simulink library "sm_wheel_loader_lib"  (R2026a)
settings: Solver=VariableStepAuto
undefined symbols (not defined in the file): AToTOrificeVector, BiPOrificeVector, boomHEArea, boomREArea, BToTOrificeVector, fluids, GRake, GToothL, GToothR, HMPST, HydFcnParams, logLoad, Position, PToAOrificeVector, PToBOrificeVector, RakeL, RakeR, testInput, Wheel_Loader, X, Y, Z
libraries: sm_lib x694, fl_lib x183, nesl_utility x74, SimscapeFluids_lib x62, sdl_lib x25, cvt_components_lib x25, simulink_extras x5, $bdroot x4, wheel_loader_contact_lib x4, ee_lib x2, SignalEditorBlockLib x1, batteryecm_lib x1
(part 3 of 25)

== system sm_wheel_loader_lib/CVT Power Split Hydromechanical/Hydrostatic ==
  Ctrl : Inport
  CV Charge Pump : fl_lib/Isothermal Liquid/Elements/Constant Volume Chamber (IL)  volume=1e-4 m^3  p_I_specify=off  p_I_priority=High  p_I=0.101325 MPa  p_I_nominal_specify=off  p_I_nominal_value=1  p_I_nominal_unit=MPa
  CV Motor A : fl_lib/Isothermal Liquid/Elements/Constant Volume Chamber (IL)  volume=1e-4 m^3  p_I_specify=off  p_I_priority=High  p_I=0.101325 MPa  p_I_nominal_specify=off  p_I_nominal_value=1  p_I_nominal_unit=MPa
  CV Motor B : fl_lib/Isothermal Liquid/Elements/Constant Volume Chamber (IL)  volume=1e-4 m^3  p_I_specify=off  p_I_priority=High  p_I=0.101325 MPa  p_I_nominal_specify=off  p_I_nominal_value=1  p_I_nominal_unit=MPa
  CV Pump A : fl_lib/Isothermal Liquid/Elements/Constant Volume Chamber (IL)  volume=1e-4 m^3  p_I_specify=off  p_I_priority=High  p_I=0.101325 MPa  p_I_nominal_specify=off  p_I_nominal_value=1  p_I_nominal_unit=MPa
  CV Pump B : fl_lib/Isothermal Liquid/Elements/Constant Volume Chamber (IL)  volume=1e-4 m^3  p_I_specify=off  p_I_priority=High  p_I=0.101325 MPa  p_I_nominal_specify=off  p_I_nominal_value=1  p_I_nominal_unit=MPa
  Charge Pump : Subsystem  Tag=PublishSubsystem  mask{chgPumpNomDisp=chgPumpNomDisp, chgPumpNomSpd=chgPumpNomSpd, chgPumpNomPressGain=chgPumpNomPressGain, chgPumpNomVolEff=chgPumpNomVolEff, chgPumpNomMechEff=chgPumpNomMechEff, chgPumpChkvPdiff=chgPumpChkvPdiff, chgPumpChkvPrange=chgPumpChkvPrange, chgPumpChkvAmax=chgPumpChkvAmax, chgPumpChkvAleak=chgPumpChkvAleak}
      mask prompts: chgPumpNomDisp "Displacement (cm^3/rev)"; chgPumpNomSpd "Nominal Angular Velocity (rpm)"; chgPumpNomPressGain "Nominal pressure gain (MPa)"; chgPumpNomVolEff "Nominal Volumetric Efficiency (0-1)"; chgPumpNomMechEff "Nominal Mechanical Efficiency (0-1)"; chgPumpChkvPdiff "Set pressure differential (MPa)"; chgPumpChkvPrange "Pressure regulation range (MPa)"; chgPumpChkvAmax "Maximum opening area (m^2)"; chgPumpChkvAleak "Leakage area (m^2)"
      mask TypeOptions chgPumpNomDisp: Pump/displacement
      mask TypeOptions chgPumpNomSpd: Pump/omega_nominal
      mask TypeOptions chgPumpNomPressGain: Pump/p_nominal
      mask TypeOptions chgPumpNomVolEff: Pump/vol_eff_nominal
      mask TypeOptions chgPumpNomMechEff: Pump/mech_eff_nominal
      mask TypeOptions chgPumpChkvPdiff:
      | Pressure
      | Relief
      | Valve/p_set_differential
      mask TypeOptions chgPumpChkvPrange:
      | Pressure
      | Relief
      | Valve/p_range
      mask TypeOptions chgPumpChkvAmax:
      | Pressure
      | Relief
      | Valve/area_max
      mask TypeOptions chgPumpChkvAleak:
      | Pressure
      | Relief
      | Valve/area_leak
      mask DialogControl grp_chg_pump Prompt: Pump
      mask DialogControl grp_chg_pump_prv Prompt: Pressure Relief Valve
      mask Display:
      | % Circle
      | color('green')
      | plot(2*cos(linspace(0, 2*pi, 100)), 2*sin(linspace(0, 2*pi, 100)))
      | % Triangle
      | patch([1 0.4 0.4]*2, [0,-0.4,0.4]*2,[45 48 173]/255)
      | % Boundary
      | color('white')
      | plot(-2, -2)
      | plot(2, 2)
  Check Valve A : SimscapeFluids_lib/Isothermal Liquid/Valves & Orifices/Directional Control Valves/Check Valve (IL)  opening_spec=2*(fluids.isothermal_liquid.valves_orifices.enum.PressureOpeningSpec.Linear)-1  pressure_control_spec=fluids.isothermal_liquid.valves_orifices.enum.pressure_control_spec.dp  p_crack_differential=p_crack_differential MPa  p_crack_gauge=0.1 MPa  press_max_differential=press_max_differential MPa  press_max_gauge=0.2 MPa  area_max=chkv_area_max m^2  area_leak=chkv_area_leak m^2  p_diff_TLU=[0.01 : 0.01 : 0.1] MPa  valve_area_TLU=[1e-10, 1e-05, 2e-05, 3e-05, 4e-05, 5e-05, 6e-05, 7.5e-05, 8.5e-05, .0001] m^2  vol_flow_TLU=[.000358, .045, .11, .191, .284, .39, .505, .63, .764, .905] .* 1e-3 m^3/s  area=inf m^2  Cd=0.64  Re_c=150  smoothing_factor=0.01  pressure_recovery=simscape.enum.onoff.off  opening_dynamics=simscape.enum.onoff.off  tau=0.1 s
  Check Valve B : SimscapeFluids_lib/Isothermal Liquid/Valves & Orifices/Directional Control Valves/Check Valve (IL)  opening_spec=2*(fluids.isothermal_liquid.valves_orifices.enum.PressureOpeningSpec.Linear)-1  pressure_control_spec=fluids.isothermal_liquid.valves_orifices.enum.pressure_control_spec.dp  p_crack_differential=p_crack_differential MPa  p_crack_gauge=0.1 MPa  press_max_differential=press_max_differential MPa  press_max_gauge=0.2 MPa  area_max=chkv_area_max m^2  area_leak=chkv_area_leak m^2  p_diff_TLU=[0.01 : 0.01 : 0.1] MPa  valve_area_TLU=[1e-10, 1e-05, 2e-05, 3e-05, 4e-05, 5e-05, 6e-05, 7.5e-05, 8.5e-05, .0001] m^2  vol_flow_TLU=[.000358, .045, .11, .191, .284, .39, .505, .63, .764, .905] .* 1e-3 m^3/s  area=inf m^2  Cd=0.64  Re_c=150  smoothing_factor=0.01  pressure_recovery=simscape.enum.onoff.off  opening_dynamics=simscape.enum.onoff.off  tau=0.1 s
  Gain1 : Gain  Gain=pumpNomDisp
  Gain2 : Gain  Gain=-1
  Mechanical Rotational Reference : fl_lib/Mechanical/Rotational Elements/Mechanical Rotational Reference
  Mechanical Rotational Reference1 : fl_lib/Mechanical/Rotational Elements/Mechanical Rotational Reference
  Motor : SimscapeFluids_lib/Isothermal Liquid/Pumps & Motors/Fixed-Displacement Motor (IL)  leakage_friction_spec=fluids.isothermal_liquid.pumps_motors.enum.MotorLossSpec.Analytical  displacement=motorNomDisp cm^3/rev  omega_nominal=motorNomSpd rpm  p_nominal=motorNomPressDrop MPa  vol_eff_nominal=motorNomVolEff  mech_eff_nominal=motorNomMechEff  no_load_torque=0 N*m  p_diff_eff_TLU=[.1, 1, 2] MPa  omega_eff_TLU=[25, 50, 100, 200, 300, 400] rad/s  vol_eff_TLU=[.816, .908, .954, .977, .981, .984; .325, .663, .831, .916, .925, .946; .137, .568, .78, .892, .893, .91]  mech_eff_TLU=[.996, .996, .996, .996, .996, .996; .988, .989, .989, .989, .989, .99; .981, .981, .982, .982, .983, .984]  p_diff_loss_TLU=[.1, 1, 2] MPa  omega_loss_TLU=[25, 50, 100, 200, 300, 400] rad/s  vol_loss_TLU=[.023, .023, .023, .023, .0285, .032; .0844, .0842, .0845, .084, .1125, .108; .1079, .108, .11, .108, .1605, .18] * 1e-3 m^3/s  mech_loss_TLU=[.002, .002, .002, .002, .002, .002; .0607, .0556, .0556, .0556, .0556, .0505; .1937, .1937, .1833, .1833, .1729, .1626] N*m  q_shaft_TLU=[.125, .25, .5, 1, 1.5, 2] * 1e-3 m^3/s  p_diff_shaft_TLU=[.1, 1, 2] MPa  torque_shaft_TLU=[.47, 4.72, 9.35; .47, 4.7, 9.36; .47, 4.7, 9.4; .47, 4.7, 9.41; .47, 4.7, 9.46; .47, 4.68, 9.5] N*m  omega_shaft_TLU=[205, 80, 35; 455, 330, 285; 955, 831, 780; 1950, 1830, 1780; 2940, 2775, 2680; 3940, 3780, 3640] rpm  vol_eff_min=1e-3  vol_eff_max=1  mech_eff_min=1e-3  mech_eff_max=1  pressure_threshold=1e-3 MPa  omega_threshold=10 rad/s  supplied_range_check=simscape.enum.assert.action.none  motor_mode_check=simscape.enum.assert.action.none  pressure_check=simscape.enum.assert.action.none  p_min_valid=0.101325 MPa
  Motor Leakage : Subsystem  Tag=PublishSubsystem
  "Pipe A " : fl_lib/Isothermal Liquid/Elements/Pipe (IL)  length=pipeLen m  area=pipeAreaGeo m^2  Dh=pipeAreaHydr m  length_add=4 m  roughness=15e-6 m  Re_lam=2000  Re_tur=4000  shape_factor=64  dynamic_compressibility=simscape.enum.onoff.on  inertia=simscape.enum.onoff.off  p0=0.101325 MPa  mdot0=0 kg/s
  Pipe B : fl_lib/Isothermal Liquid/Elements/Pipe (IL)  length=pipeLen m  area=pipeAreaGeo m^2  Dh=pipeAreaHydr m  length_add=4 m  roughness=15e-6 m  Re_lam=2000  Re_tur=4000  shape_factor=64  dynamic_compressibility=simscape.enum.onoff.on  inertia=simscape.enum.onoff.off  p0=0.101325 MPa  mdot0=0 kg/s
  Pressure Relief Valve A : SimscapeFluids_lib/Isothermal Liquid/Valves & Orifices/Pressure Control Valves/Pressure Relief Valve (IL)  set_pressure_spec=foundation.enum.constant_controlled.constant  opening_spec=fluids.isothermal_liquid.valves_orifices.enum.opening_spec.linear  pressure_spec=fluids.isothermal_liquid.valves_orifices.enum.pressure_control_spec.dp  p_set_gauge=0.1 MPa  p_set_differential=p_set_differential MPa  p_range=p_range MPa  area_max=prv_area_max m^2  area_leak=prv_area_leak m^2  p_diff_TLU=[0.2 : 0.2 : 1.2] MPa  p_gauge_TLU=[0.2 : 0.2 : 1.2] MPa  valve_area_TLU=[1e-10, 2e-06, 4e-06, 6e-06, 8e-06, 1e-05] m^2  vol_flow_TLU=[1e-09, 3.6e-05, 8.9e-05, .00015, .00023, .00031] m^3/s  area=inf m^2  Cd=0.64  Re_c=150  smoothing_factor=0.01  pressure_recovery=simscape.enum.onoff.off  opening_dynamics=simscape.enum.onoff.off  tau=0.1 s
  Pressure Relief Valve B : SimscapeFluids_lib/Isothermal Liquid/Valves & Orifices/Pressure Control Valves/Pressure Relief Valve (IL)  set_pressure_spec=foundation.enum.constant_controlled.constant  opening_spec=fluids.isothermal_liquid.valves_orifices.enum.opening_spec.linear  pressure_spec=fluids.isothermal_liquid.valves_orifices.enum.pressure_control_spec.dp  p_set_gauge=0.1 MPa  p_set_differential=p_set_differential MPa  p_range=p_range MPa  area_max=prv_area_max m^2  area_leak=prv_area_leak m^2  p_diff_TLU=[0.2 : 0.2 : 1.2] MPa  p_gauge_TLU=[0.2 : 0.2 : 1.2] MPa  valve_area_TLU=[1e-10, 2e-06, 4e-06, 6e-06, 8e-06, 1e-05] m^2  vol_flow_TLU=[1e-09, 3.6e-05, 8.9e-05, .00015, .00023, .00031] m^3/s  area=inf m^2  Cd=0.64  Re_c=150  smoothing_factor=0.01  pressure_recovery=simscape.enum.onoff.off  opening_dynamics=simscape.enum.onoff.off  tau=0.1 s
  Pump : SimscapeFluids_lib/Isothermal Liquid/Pumps & Motors/Variable-Displacement Pump (IL)  leakage_friction_spec=fluids.isothermal_liquid.pumps_motors.enum.pump_motor_loss_spec.analytical  displacement_nominal=pumpNomDisp cm^3/rev  omega_nominal=pumpNomSpd rpm  p_nominal=pumpNomPressGain MPa  vol_eff_nominal=pumpNomVolEff  mech_eff_nominal=pumpNomMechEff  no_load_torque=0 N*m  p_diff_eff_TLU=[.1, 1, 2] MPa  omega_eff_TLU=[25, 50, 100, 200, 300, 400] rad/s  displacement_eff_TLU=[-30, -19, 19, 30] cm^3/rev  vol_eff_TLU=repmat([.816, .908, .954, .977, .981, .984; .325, .663, .831, .916, .925, .946; .137, .568, .78, .892, .893, .91], 1, 1, 4)  mech_eff_TLU=repmat([.996, .996, .996, .996, .996, .996; .988, .989, .989, .989, .989, .99; .981, .981, .982, .982, .983, .984], 1, 1, 4)  p_diff_loss_TLU=[.1, 1, 2] MPa  omega_loss_TLU=[25, 50, 100, 200, 300, 400] rad/s  displacement_loss_TLU=[-30, -19, 19, 30] cm^3/rev  vol_loss_TLU=repmat([.023, .023, .023, .023, .0285, .032; .0844, .0842, .0845, .084, .1125, .108; .1079, .108, .11, .108, .1605, .18] * 1e-3, 1, 1, 4) m^3/s  mech_loss_TLU=repmat([.002, .002, .002, .002, .002, .002; .0607, .0556, .0556, .0556, .0556, .0505; .1937, .1937, .1833, .1833, .1729, .1626], 1, 1, 4) N*m  vol_eff_min=1e-3  vol_eff_max=1  mech_eff_min=1e-3  mech_eff_max=1  pressure_threshold=1e-3 MPa  omega_threshold=10 rad/s  displacement_threshold=0.1 cm^3/rev  supplied_range_check=simscape.enum.assert.action.none  pump_mode_check=simscape.enum.assert.action.none  pressure_check=simscape.enum.assert.action.none  p_min_valid=0.101325 MPa
  Pump Leakage : Subsystem  Tag=PublishSubsystem
  Simulink-PS Converter1 : nesl_utility/Simulink-PS Converter  PhysicalDomain=network_engine_domain  SubClassName=ps_input  LeftPortType=input  RightPortType=output  PseudoPeriodic=off  Frequencies=[]  NoiseDistribution=none  NoiseParameters=[]  Unit=cm^3/rev  AffineConversion=off  FilteringAndDerivatives=provide  SimscapeFilterOrder=1  InputFilterTimeConstant=0.001  UdotUserProvided=0
  Transmission Fluid Properties : fl_lib/Isothermal Liquid/Utilities/Isothermal Liquid Properties (IL)  rho_L_atm=850 kg/m^3  bulk_modulus_model=foundation.enum.bulk_modulus_model.const  beta_gain=6  beta_L_atm=1.4 GPa  nu_atm=18.8 cSt  p_atm=0.101325 MPa  p_min=0.1 Pa  properties_range_check=simscape.enum.assert.action.error  air_fraction=0.005  polytropic_index=1.0  rho_g_atm=1.225 kg/m^3  air_dissolution_model=simscape.enum.onoff.off  p_crit=3 MPa
  In : PMIOPort  Side=Left
  Out : PMIOPort  Port=2  Side=Right
  wires:
  Ctrl/1 -> Gain2/1
  Gain1/1 -> Simulink-PS Converter1/1
  Gain2/1 -> Gain1/1
  connections:
  In/RConn1 -- Charge Pump/LConn1 -- Pump/RConn1
  Motor/RConn1 -- Out/RConn1
  Mechanical Rotational Reference1/LConn1 -- Pump/RConn2
  Pressure Relief Valve A/LConn1 -- Pressure Relief Valve B/RConn1 -- Motor Leakage/LConn1 -- CV Motor A/LConn1 -- Motor/LConn1 -- "Pipe A "/RConn1
  Motor/RConn2 -- Mechanical Rotational Reference/LConn1
  Check Valve B/LConn1 -- Check Valve A/LConn1 -- Charge Pump/RConn1 -- CV Charge Pump/LConn1
  Check Valve A/RConn1 -- Pump Leakage/LConn1 -- Transmission Fluid Properties/RConn1 -- CV Pump B/LConn1 -- Pump/LConn2 -- "Pipe A "/LConn1
  Check Valve B/RConn1 -- Pump Leakage/LConn2 -- CV Pump A/LConn1 -- Pump/RConn3 -- Pipe B/LConn1
  Pressure Relief Valve A/RConn1 -- Pressure Relief Valve B/LConn1 -- Motor Leakage/LConn2 -- CV Motor B/LConn1 -- Motor/RConn3 -- Pipe B/RConn1
  Simulink-PS Converter1/RConn1 -- Pump/LConn1

== system sm_wheel_loader_lib/CVT Power Split Hydromechanical/Sensor P1s ==
  MRRef : fl_lib/Mechanical/Rotational Elements/Mechanical Rotational Reference
  Motion Sensor : fl_lib/Mechanical/Mechanical Sensors/Ideal Rotational Motion Sensor  reference=foundation.enum.MeasurementReference.difference  acceleration_port=false  velocity_port=true  position_port=false  wrap_angle=false  offset=0 rad
  PS-Simulink Converter : nesl_utility/PS-Simulink Converter  PhysicalDomain=network_engine_domain  SubClassName=ps_output  LeftPortType=input  RightPortType=output  PseudoPeriodic=off  Frequencies=[]  VectorFormat=inherit  Unit=rpm  AffineConversion=off
  R : PMIOPort  Side=Left
  w : Outport
  wires:
  PS-Simulink Converter/1 -> w/1
  connections:
  R/RConn1 -- Motion Sensor/LConn1
  MRRef/LConn1 -- Motion Sensor/RConn1
  PS-Simulink Converter/LConn1 -- Motion Sensor/RConn2

== system sm_wheel_loader_lib/CVT Power Split Hydromechanical/Sensor wG2 ==
  MRRef : fl_lib/Mechanical/Rotational Elements/Mechanical Rotational Reference
  Motion Sensor : fl_lib/Mechanical/Mechanical Sensors/Ideal Rotational Motion Sensor  reference=foundation.enum.MeasurementReference.difference  acceleration_port=false  velocity_port=true  position_port=false  wrap_angle=false  offset=0 rad
  PS-Simulink Converter : nesl_utility/PS-Simulink Converter  PhysicalDomain=network_engine_domain  SubClassName=ps_output  LeftPortType=input  RightPortType=output  PseudoPeriodic=off  Frequencies=[]  VectorFormat=inherit  Unit=rpm  AffineConversion=off
  R : PMIOPort  Side=Left
  w : Outport
  wires:
  PS-Simulink Converter/1 -> w/1
  connections:
  R/RConn1 -- Motion Sensor/LConn1
  MRRef/LConn1 -- Motion Sensor/RConn1
  PS-Simulink Converter/LConn1 -- Motion Sensor/RConn2

== system sm_wheel_loader_lib/CVT Power Split Hydromechanical/Sensor wG3 ==
  MRRef : fl_lib/Mechanical/Rotational Elements/Mechanical Rotational Reference
  Motion Sensor : fl_lib/Mechanical/Mechanical Sensors/Ideal Rotational Motion Sensor  reference=foundation.enum.MeasurementReference.difference  acceleration_port=false  velocity_port=true  position_port=false  wrap_angle=false  offset=0 rad
  PS-Simulink Converter : nesl_utility/PS-Simulink Converter  PhysicalDomain=network_engine_domain  SubClassName=ps_output  LeftPortType=input  RightPortType=output  PseudoPeriodic=off  Frequencies=[]  VectorFormat=inherit  Unit=rpm  AffineConversion=off
  R : PMIOPort  Side=Left
  w : Outport
  wires:
  PS-Simulink Converter/1 -> w/1
  connections:
  PS-Simulink Converter/LConn1 -- Motion Sensor/RConn2
  MRRef/LConn1 -- Motion Sensor/RConn1
  R/RConn1 -- Motion Sensor/LConn1

== system sm_wheel_loader_lib/CVT Power Split Hydromechanical/Sensor wG4 ==
  MRRef : fl_lib/Mechanical/Rotational Elements/Mechanical Rotational Reference
  Motion Sensor : fl_lib/Mechanical/Mechanical Sensors/Ideal Rotational Motion Sensor  reference=foundation.enum.MeasurementReference.difference  acceleration_port=false  velocity_port=true  position_port=false  wrap_angle=false  offset=0 rad
  PS-Simulink Converter : nesl_utility/PS-Simulink Converter  PhysicalDomain=network_engine_domain  SubClassName=ps_output  LeftPortType=input  RightPortType=output  PseudoPeriodic=off  Frequencies=[]  VectorFormat=inherit  Unit=rpm  AffineConversion=off
  R : PMIOPort  Side=Left
  w : Outport
  wires:
  PS-Simulink Converter/1 -> w/1
  connections:
  PS-Simulink Converter/LConn1 -- Motion Sensor/RConn2
  MRRef/LConn1 -- Motion Sensor/RConn1
  R/RConn1 -- Motion Sensor/LConn1

== system sm_wheel_loader_lib/CVT Power Split Hydromechanical/Sensor wIn ==
  MRRef : fl_lib/Mechanical/Rotational Elements/Mechanical Rotational Reference
  Motion Sensor : fl_lib/Mechanical/Mechanical Sensors/Ideal Rotational Motion Sensor  reference=foundation.enum.MeasurementReference.difference  acceleration_port=false  velocity_port=true  position_port=false  wrap_angle=false  offset=0 rad
  PS-Simulink Converter : nesl_utility/PS-Simulink Converter  PhysicalDomain=network_engine_domain  SubClassName=ps_output  LeftPortType=input  RightPortType=output  PseudoPeriodic=off  Frequencies=[]  VectorFormat=inherit  Unit=rpm  AffineConversion=off
  R : PMIOPort  Side=Left
  w : Outport
  wires:
  PS-Simulink Converter/1 -> w/1
  connections:
  PS-Simulink Converter/LConn1 -- Motion Sensor/RConn2
  MRRef/LConn1 -- Motion Sensor/RConn1
  R/RConn1 -- Motion Sensor/LConn1

== system sm_wheel_loader_lib/CVT Power Split Hydromechanical/Sensor wOut ==
  MRRef : fl_lib/Mechanical/Rotational Elements/Mechanical Rotational Reference
  Motion Sensor : fl_lib/Mechanical/Mechanical Sensors/Ideal Rotational Motion Sensor  reference=foundation.enum.MeasurementReference.difference  acceleration_port=false  velocity_port=true  position_port=false  wrap_angle=false  offset=0 rad
  PS-Simulink Converter : nesl_utility/PS-Simulink Converter  PhysicalDomain=network_engine_domain  SubClassName=ps_output  LeftPortType=input  RightPortType=output  PseudoPeriodic=off  Frequencies=[]  VectorFormat=inherit  Unit=rpm  AffineConversion=off
  R : PMIOPort  Side=Left
  w : Outport
  wires:
  PS-Simulink Converter/1 -> w/1
  connections:
  R/RConn1 -- Motion Sensor/LConn1
  MRRef/LConn1 -- Motion Sensor/RConn1
  PS-Simulink Converter/LConn1 -- Motion Sensor/RConn2

== system sm_wheel_loader_lib/CVT Power Split Hydromechanical/Sensor wP1c ==
  MRRef : fl_lib/Mechanical/Rotational Elements/Mechanical Rotational Reference
  Motion Sensor : fl_lib/Mechanical/Mechanical Sensors/Ideal Rotational Motion Sensor  reference=foundation.enum.MeasurementReference.difference  acceleration_port=false  velocity_port=true  position_port=false  wrap_angle=false  offset=0 rad
  PS-Simulink Converter : nesl_utility/PS-Simulink Converter  PhysicalDomain=network_engine_domain  SubClassName=ps_output  LeftPortType=input  RightPortType=output  PseudoPeriodic=off  Frequencies=[]  VectorFormat=inherit  Unit=rpm  AffineConversion=off
  R : PMIOPort  Side=Left
  w : Outport
  wires:
  PS-Simulink Converter/1 -> w/1
  connections:
  R/RConn1 -- Motion Sensor/LConn1
  MRRef/LConn1 -- Motion Sensor/RConn1
  PS-Simulink Converter/LConn1 -- Motion Sensor/RConn2

== system sm_wheel_loader_lib/CVT Power Split Hydromechanical/Sensor wP2s ==
  MRRef : fl_lib/Mechanical/Rotational Elements/Mechanical Rotational Reference
  Motion Sensor : fl_lib/Mechanical/Mechanical Sensors/Ideal Rotational Motion Sensor  reference=foundation.enum.MeasurementReference.difference  acceleration_port=false  velocity_port=true  position_port=false  wrap_angle=false  offset=0 rad
  PS-Simulink Converter : nesl_utility/PS-Simulink Converter  PhysicalDomain=network_engine_domain  SubClassName=ps_output  LeftPortType=input  RightPortType=output  PseudoPeriodic=off  Frequencies=[]  VectorFormat=inherit  Unit=rpm  AffineConversion=off
  R : PMIOPort  Side=Left
  w : Outport
  wires:
  PS-Simulink Converter/1 -> w/1
  connections:
  PS-Simulink Converter/LConn1 -- Motion Sensor/RConn2
  MRRef/LConn1 -- Motion Sensor/RConn1
  R/RConn1 -- Motion Sensor/LConn1

== system sm_wheel_loader_lib/CVT Power Split Hydromechanical/Sensor wP3r ==
  MRRef : fl_lib/Mechanical/Rotational Elements/Mechanical Rotational Reference
  Motion Sensor : fl_lib/Mechanical/Mechanical Sensors/Ideal Rotational Motion Sensor  reference=foundation.enum.MeasurementReference.difference  acceleration_port=false  velocity_port=true  position_port=false  wrap_angle=false  offset=0 rad
  PS-Simulink Converter : nesl_utility/PS-Simulink Converter  PhysicalDomain=network_engine_domain  SubClassName=ps_output  LeftPortType=input  RightPortType=output  PseudoPeriodic=off  Frequencies=[]  VectorFormat=inherit  Unit=rpm  AffineConversion=off
  R : PMIOPort  Side=Left
  w : Outport
  wires:
  PS-Simulink Converter/1 -> w/1
  connections:
  PS-Simulink Converter/LConn1 -- Motion Sensor/RConn2
  MRRef/LConn1 -- Motion Sensor/RConn1
  R/RConn1 -- Motion Sensor/LConn1

== system sm_wheel_loader_lib/CVT Power Split Hydromechanical/Sensor wP4c ==
  MRRef : fl_lib/Mechanical/Rotational Elements/Mechanical Rotational Reference
  Motion Sensor : fl_lib/Mechanical/Mechanical Sensors/Ideal Rotational Motion Sensor  reference=foundation.enum.MeasurementReference.difference  acceleration_port=false  velocity_port=true  position_port=false  wrap_angle=false  offset=0 rad
  PS-Simulink Converter : nesl_utility/PS-Simulink Converter  PhysicalDomain=network_engine_domain  SubClassName=ps_output  LeftPortType=input  RightPortType=output  PseudoPeriodic=off  Frequencies=[]  VectorFormat=inherit  Unit=rpm  AffineConversion=off
  R : PMIOPort  Side=Left
  w : Outport
  wires:
  PS-Simulink Converter/1 -> w/1
  connections:
  PS-Simulink Converter/LConn1 -- Motion Sensor/RConn2
  MRRef/LConn1 -- Motion Sensor/RConn1
  R/RConn1 -- Motion Sensor/LConn1

== system sm_wheel_loader_lib/CVT Power Split Hydromechanical/Sensor wP4r ==
  MRRef : fl_lib/Mechanical/Rotational Elements/Mechanical Rotational Reference
  Motion Sensor : fl_lib/Mechanical/Mechanical Sensors/Ideal Rotational Motion Sensor  reference=foundation.enum.MeasurementReference.difference  acceleration_port=false  velocity_port=true  position_port=false  wrap_angle=false  offset=0 rad
  PS-Simulink Converter : nesl_utility/PS-Simulink Converter  PhysicalDomain=network_engine_domain  SubClassName=ps_output  LeftPortType=input  RightPortType=output  PseudoPeriodic=off  Frequencies=[]  VectorFormat=inherit  Unit=rpm  AffineConversion=off
  R : PMIOPort  Side=Left
  w : Outport
  wires:
  PS-Simulink Converter/1 -> w/1
  connections:
  R/RConn1 -- Motion Sensor/LConn1
  MRRef/LConn1 -- Motion Sensor/RConn1
  PS-Simulink Converter/LConn1 -- Motion Sensor/RConn2

== system sm_wheel_loader_lib/CVT Power Split Hydromechanical/Sensor wP4s ==
  MRRef : fl_lib/Mechanical/Rotational Elements/Mechanical Rotational Reference
  Motion Sensor : fl_lib/Mechanical/Mechanical Sensors/Ideal Rotational Motion Sensor  reference=foundation.enum.MeasurementReference.difference  acceleration_port=false  velocity_port=true  position_port=false  wrap_angle=false  offset=0 rad
  PS-Simulink Converter : nesl_utility/PS-Simulink Converter  PhysicalDomain=network_engine_domain  SubClassName=ps_output  LeftPortType=input  RightPortType=output  PseudoPeriodic=off  Frequencies=[]  VectorFormat=inherit  Unit=rpm  AffineConversion=off
  R : PMIOPort  Side=Left
  w : Outport
  wires:
  PS-Simulink Converter/1 -> w/1
  connections:
  PS-Simulink Converter/LConn1 -- Motion Sensor/RConn2
  MRRef/LConn1 -- Motion Sensor/RConn1
  R/RConn1 -- Motion Sensor/LConn1

== system sm_wheel_loader_lib/Controller/CVT Ratio Ctrl ==
  Ratio (-) : Inport
  CmdVehSpdDir : Inport  Port=2
  HRBCtrl (-) : Inport  Port=3
  MBCtrl (-) : Inport  Port=4
  Bus Creator : BusCreator  Inputs=12
  Clutch Truth Table : Stateflow chart  TreatAsAtomicUnit=on
  Filter : StateSpace  A=-200  C=200  D=0  InitialCondition=HMPST.Ctrl.Swash.XY_A(1,1)/200
  Range Calculation : Subsystem  mask{XY_I=HMPST.Ctrl.Swash.XY_I}
      mask prompts: XY_I "Range Separation Points"
  Saturation : Saturate  UpperLimit=HMPST.DesignReq.MaxCVTOutputSpeed/HMPST.Eng.wTarget  LowerLimit=0  ZeroCross=off
  Swash Ctrl : Lookup_n-D  NumberOfTableDimensions=1  BreakpointsForDimension1=HMPST.Ctrl.Swash.XY_A(:,2)  BeginIndexSearchUsingPreviousIndexResult=on  Table=HMPST.Ctrl.Swash.XY_A(:,1)  InternalRulePriority=Speed  RndMeth=Simplest
  Transfer Fcn : TransferFcn  Denominator=[0.1 1]
  CVT Ctrl : Outport
  wires:
  Ratio (-)/1 -> [ratio], Transfer Fcn/1
  Clutch Truth Table/1(K1Actv) -> Bus Creator/1  "K1"
  Clutch Truth Table/2(K2Actv) -> Bus Creator/2  "K2"
  Clutch Truth Table/3(K3Actv) -> Bus Creator/3  "K3"
  Clutch Truth Table/4(K4Actv) -> Bus Creator/4  "K4"
  Clutch Truth Table/5(KbActv) -> Bus Creator/5  "Kb"
  Clutch Truth Table/6(KvActv) -> Bus Creator/6  "Kv"
  Clutch Truth Table/7(KrActv) -> Bus Creator/7  "Kr"
  Bus Creator/1 -> CVT Ctrl/1  "Ctrl"
  Range Calculation/1(Range (-)) -> Clutch Truth Table/1(Range)
  Saturation/1 -> Swash Ctrl/1, Range Calculation/1(Ratio (-))
  Transfer Fcn/1 -> Saturation/1
  Filter/1 -> Bus Creator/12  "SwashCtrl"
  Swash Ctrl/1 -> Filter/1  "SwashCtrl"
  HRBCtrl (-)/1 -> Bus Creator/8  "HRBCtrl"
  MBCtrl (-)/1 -> Bus Creator/9  "MBCtrl"
  CmdVehSpdDir/1 -> Bus Creator/11, Clutch Truth Table/2(CmdVehSpdDir)  "CmdVehSpdDir"
  [ratio] -> Bus Creator/10  "ratio"

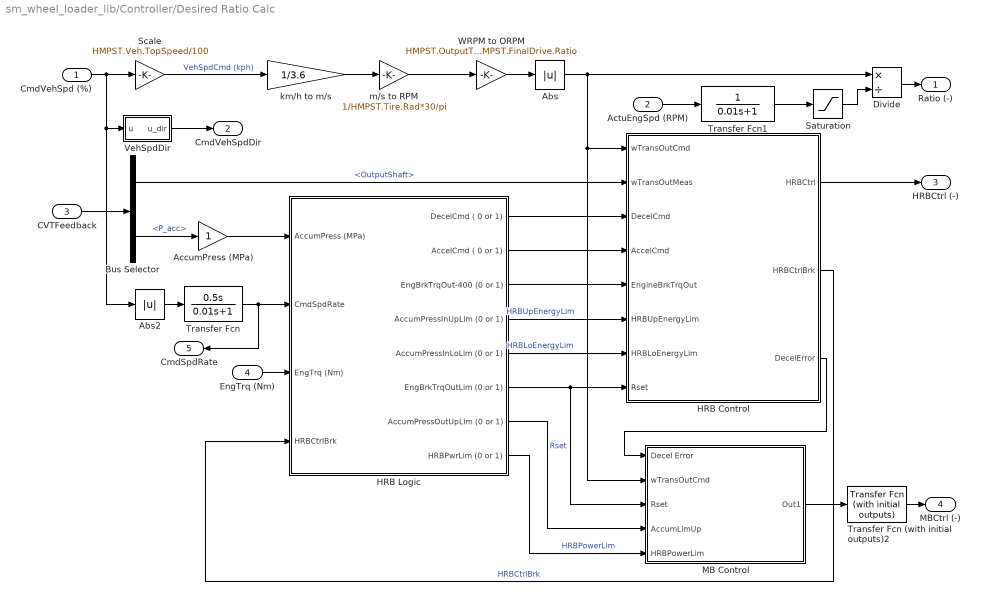
== system sm_wheel_loader_lib/Controller/Desired Ratio Calc ==
  CmdVehSpd (%) : Inport  SampleTime=HMPST.Simu.TimeStep
  ActuEngSpd (RPM) : Inport  Port=2
  CVTFeedback : Inport  Port=3
  EngTrq (Nm) : Inport  Port=4
  Abs : Abs  ZeroCross=off  SaturateOnIntegerOverflow=off
  Abs2 : Abs  ZeroCross=off  SaturateOnIntegerOverflow=off
  AccumPress (MPa) : Gain
  Bus Selector : BusSelector  OutputSignals=OutputShaft,P_acc
  Divide : Product  Inputs=*/
  HRB Control : Subsystem
  HRB Logic : Subsystem
  MB Control : Subsystem
  Saturation : Saturate  UpperLimit=2500  LowerLimit=0.5
  Scale : Gain  Gain=HMPST.Veh.TopSpeed/100
  Transfer Fcn : TransferFcn  Numerator=[0.5 0]  Denominator=[0.01 1]
  Transfer Fcn (with initial outputs)2 : simulink_extras/Additional Linear/Transfer Fcn (with initial outputs)  N=1  D=[0.05 1]  Y0=1  U0=1
  Transfer Fcn1 : TransferFcn  Denominator=[0.01 1]
  VehSpdDir : Subsystem
  WRPM to ORPM : Gain  Gain=HMPST.OutputTransferGearPair.Ratio*HMPST.Differential.Ratio*HMPST.FinalDrive.Ratio
  km/h to m/s : Gain  Gain=1/3.6
  m/s to RPM : Gain  Gain=1/HMPST.Tire.Rad*30/pi
  Ratio (-) : Outport
  CmdVehSpdDir : Outport  Port=2
  HRBCtrl (-) : Outport  Port=3
  MBCtrl (-) : Outport  Port=4
  CmdSpdRate : Outport  Port=5
  wires:
  MB Control/1(Out1) -> Transfer Fcn (with initial outputs)2/1
  HRB Logic/8(HRBPwrLim (0 or 1)) -> MB Control/5(HRBPowerLim)  "HRBPowerLim"
  HRB Logic/7(AccumPressOutUpLim (0 or 1)) -> MB Control/4(AccumLimUp)
  HRB Control/3(DecelError) -> MB Control/1(Decel Error)
  HRB Control/1(HRBCtrl) -> HRBCtrl (-)/1
  HRB Logic/3(EngBrkTrqOut-400 (0 or 1)) -> HRB Control/5(EngineBrkTrqOut)
  HRB Logic/2(AccelCmd ( 0 or 1)) -> HRB Control/4(AccelCmd)
  HRB Logic/5(AccumPressInLoLim (0 or 1)) -> HRB Control/7(HRBLoEnergyLim)  "HRBLoEnergyLim"
  HRB Logic/4(AccumPressInUpLim (0 or 1)) -> HRB Control/6(HRBUpEnergyLim)  "HRBUpEnergyLim"
  HRB Logic/1(DecelCmd ( 0 or 1)) -> HRB Control/3(DecelCmd)
  Divide/1 -> Ratio (-)/1
  ActuEngSpd (RPM)/1 -> Transfer Fcn1/1
  m/s to RPM/1 -> WRPM to ORPM/1
  km/h to m/s/1 -> m/s to RPM/1
  WRPM to ORPM/1 -> Abs/1
  CmdVehSpd (%)/1 -> Abs2/1, VehSpdDir/1(u), Scale/1
  Saturation/1 -> Divide/2
  Transfer Fcn1/1 -> Saturation/1
  Bus Selector/1 -> HRB Control/2(wTransOutMeas)  "<OutputShaft>"
  Transfer Fcn/1 -> HRB Logic/2(CmdSpdRate), CmdSpdRate/1
  CVTFeedback/1 -> Bus Selector/1
  HRB Logic/6(EngBrkTrqOutLim (0 or 1)) -> MB Control/3(Rset), HRB Control/8(Rset)  "Rset"
  Bus Selector/2 -> AccumPress (MPa)/1  "<P_acc>"
  EngTrq (Nm)/1 -> HRB Logic/3(EngTrq (Nm))
  AccumPress (MPa)/1 -> HRB Logic/1(AccumPress (MPa))
  VehSpdDir/1(u_dir) -> CmdVehSpdDir/1
  Scale/1 -> km/h to m/s/1  "VehSpdCmd (kph)"
  Abs2/1 -> Transfer Fcn/1
  Abs/1 -> Divide/1, MB Control/2(wTransOutCmd), HRB Control/1(wTransOutCmd)
  Transfer Fcn (with initial outputs)2/1 -> MBCtrl (-)/1
  HRB Control/2(HRBCtrlBrk) -> HRB Logic/4(HRBCtrlBrk)  "HRBCtrlBrk"

== system sm_wheel_loader_lib/Engine Droop/Speed Sensor ==
  MRRef : fl_lib/Mechanical/Rotational Elements/Mechanical Rotational Reference
  Motion Sensor : fl_lib/Mechanical/Mechanical Sensors/Ideal Rotational Motion Sensor  reference=foundation.enum.MeasurementReference.difference  acceleration_port=false  velocity_port=true  position_port=false  wrap_angle=false  offset=0 rad
  Press A3 : nesl_utility/PS-Simulink Converter  PhysicalDomain=network_engine_domain  SubClassName=ps_output  LeftPortType=input  RightPortType=output  PseudoPeriodic=off  Frequencies=[]  VectorFormat=1-D array  Unit=rpm  AffineConversion=off
  Transfer Fcn : TransferFcn  Denominator=[0.1 1]
  R : PMIOPort  Side=Left
  rpm : Outport
  wires:
  Transfer Fcn/1 -> rpm/1
  Press A3/1 -> Transfer Fcn/1
  connections:
  R/RConn1 -- Motion Sensor/LConn1
  MRRef/LConn1 -- Motion Sensor/RConn1
  Motion Sensor/RConn2 -- Press A3/LConn1

== system sm_wheel_loader_lib/Engine Droop/Torque Sensor ==
  PS-Simulink Converter : nesl_utility/PS-Simulink Converter  PhysicalDomain=network_engine_domain  SubClassName=ps_output  LeftPortType=input  RightPortType=output  PseudoPeriodic=off  Frequencies=[]  VectorFormat=inherit  Unit=inherit  AffineConversion=off
  Torque Sensor : fl_lib/Mechanical/Mechanical Sensors/Ideal Torque Sensor
  R : PMIOPort  Side=Left
  C : PMIOPort  Port=2  Side=Right
  m : Outport
  wires:
  PS-Simulink Converter/1 -> m/1
  connections:
  PS-Simulink Converter/LConn1 -- Torque Sensor/RConn2
  Torque Sensor/LConn1 -- R/RConn1
  C/RConn1 -- Torque Sensor/RConn1

== system sm_wheel_loader_lib/Engine Generic/Speed Sensor ==
  Ideal Rotational Motion Sensor1 : fl_lib/Mechanical/Mechanical Sensors/Ideal Rotational Motion Sensor  reference=foundation.enum.MeasurementReference.difference  acceleration_port=false  velocity_port=true  position_port=false  wrap_angle=false  offset=0 rad
  Mechanical Rotational Reference1 : fl_lib/Mechanical/Rotational Elements/Mechanical Rotational Reference
  Press A3 : nesl_utility/PS-Simulink Converter  PhysicalDomain=network_engine_domain  SubClassName=ps_output  LeftPortType=input  RightPortType=output  PseudoPeriodic=off  Frequencies=[]  VectorFormat=1-D array  Unit=rpm  AffineConversion=off
  Transfer Fcn : TransferFcn  Denominator=[0.1 1]
  R : PMIOPort  Side=Left
  w (rpm) : Outport
  wires:
  Transfer Fcn/1 -> w (rpm)/1
  Press A3/1 -> Transfer Fcn/1
  connections:
  R/RConn1 -- Ideal Rotational Motion Sensor1/LConn1
  Mechanical Rotational Reference1/LConn1 -- Ideal Rotational Motion Sensor1/RConn1
  Ideal Rotational Motion Sensor1/RConn2 -- Press A3/LConn1

== system sm_wheel_loader_lib/Engine Generic/Subsystem ==
  Ideal Torque Sensor : fl_lib/Mechanical/Mechanical Sensors/Ideal Torque Sensor
  PS-Simulink Converter : nesl_utility/PS-Simulink Converter  PhysicalDomain=network_engine_domain  SubClassName=ps_output  LeftPortType=input  RightPortType=output  PseudoPeriodic=off  Frequencies=[]  VectorFormat=inherit  Unit=inherit  AffineConversion=off
  R : PMIOPort  Side=Left
  C : PMIOPort  Port=2  Side=Right
  m : Outport
  wires:
  PS-Simulink Converter/1 -> m/1
  connections:
  PS-Simulink Converter/LConn1 -- Ideal Torque Sensor/RConn2
  Ideal Torque Sensor/LConn1 -- R/RConn1
  C/RConn1 -- Ideal Torque Sensor/RConn1

== system sm_wheel_loader_lib/Wheel Loader Vehicle/Actuators ==
  Cmd : Inport
  pwr : Inport  Port=2
  Hydraulic : Subsystem  VariantControl=Hydraulic  mask{popup_impl=Bucket}
      mask prompts: popup_impl "Implement"
      mask init:
      | if(strcmp(get_param(gcb,'popup_impl'),'Bucket'))
      |     set_param([gcb '/Implement'],'LabelModeActiveChoice','Bucket');
      | else
      |     set_param([gcb '/Implement'],'LabelModeActiveChoice','Grapple');
      | end
      mask TypeOptions popup_impl: Bucket | Grapple
      mask Display: image('sm_wheel_loader_actuators_hydraulic_IMAGE.png')
  Ideal : Subsystem  VariantControl=Ideal
      mask Display: image('sm_wheel_loader_actuators_ideal_IMAGE.png')
  LiftL : PMIOPort  Side=Right
  LiftR : PMIOPort  Port=2  Side=Right
  PTO : PMIOPort  Port=3  Side=Left
  RTilt : PMIOPort  Port=4  Side=Left
  Impl : PMIOPort  Port=5  Side=Right
  Steer : PMIOPort  Port=6  Side=Right
  SWhl : PMIOPort  Port=7  Side=Left

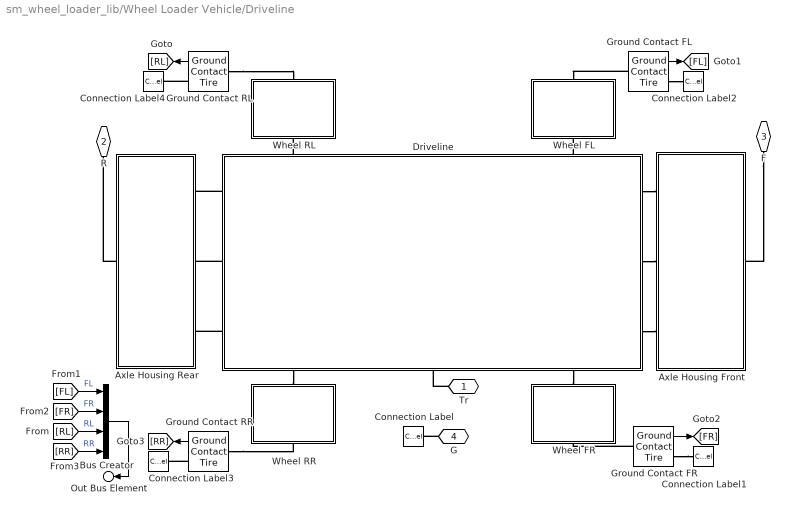
== system sm_wheel_loader_lib/Wheel Loader Vehicle/Driveline ==
  Axle Housing Front : Subsystem  Tag=26328293-4415-CB41-A9FB-B9AA4EE664BB  mask{fa_casing_opc=HMPST.Vis.FAxleHou.opc}
      mask prompts: fa_casing_opc "Casing Opacity"
      mask Display: image('sm_wheel_loader_Driveline3D_FAxleHou_IMAGE.png')
  Axle Housing Rear : Subsystem  Tag=1D918CE5-F562-3F48-9394-464191D609BF  mask{ra_casing_opc=HMPST.Vis.RAxleHou.opc}
      mask prompts: ra_casing_opc "Casing Opacity (0-1)"
      mask Display: image('sm_wheel_loader_Driveline3D_RAxleHou_IMAGE.png')
  Bus Creator : BusCreator  Inputs=4
  Connection Label{,1..4} (5 alike) : ConnectionLabel  Label=G
  Driveline : Subsystem  Variant=on  VariantControlMode=label  VariantControl=Choice  LabelModeActiveChoice=Driveline_1D  mask{popup_driveJointF=CV Joint, popup_driveJointR=CV Joint}
      mask prompts: popup_driveJointF "Driveshaft Joint (front)"; popup_driveJointR "Driveshaft Joint (rear)"
      mask init:
      | if(strcmp(get_param(gcb,'popup_driveJointF'),'CV Joint'))
      |     set_param([gcb '/Driveline 3D'],'popup_driveJointF','CV Joint')
      | else
      |     set_param([gcb '/Driveline 3D'],'popup_driveJointF','U Joint')
      | end
      | if(strcmp(get_param(gcb,'popup_driveJointR'),'CV Joint'))
      |     set_param([gcb '/Driveline 3D'],'popup_driveJointR','CV Joint')
      | else
      |     set_param([gcb '/Driveline 3D'],'popup_driveJointR','U Joint')
      | end
      settings: AttributesFormatString=%<LabelModeActiveChoice>  PortSchema="{\"entries\":[{\"content\":{\"sides\":[{\"content\":{\"connectorIds\":[\"LConn1\",\"LConn2\",\"LConn3\"]},\"type\":\"ConnectorPlacement.EquallySpacedRectSide\",\"uuid\":\"ac94f403-7500-4d3b-9e0f-075c8f20a849\"},{\"content\":{\"connectorIds\":[\"RConn1\",\"RConn2\",\"RConn3\"],\"side\":\"RIGHT\"},\"type\":\"ConnectorPlacement.EquallySpacedRectSide\",\"uuid\":\"0eb844aa-00af-4edc-a570-50ab4e6b66c2\"},{\"content\":{\"connectorIds\":[\"LConn4\",\"LConn5\",\"LConn6\"],\"side\":\"TOP\"},\"type\":\"ConnectorPlacement.EquallySpacedRectSide\",\"uuid\":\"abddfcb0-9899-4667-9404-ac15e4716921\"},{\"content\":{\"connectorIds\":[\"RConn4\",\"RConn5\",\"RConn6\"],\"side\":\"BOTTOM\"},\"type\":\"ConnectorPlacement.EquallySpacedRectSide\",\"uuid\":\"a33fa760-6818-409d-ace3-b40bc7e3acff\"}]},\"type\":\"ConnectorPlacement.EquallySpacedConnector\",\"uuid\":\"2bc03850-1261-46ce-b9b6-2dbda85e9fb0\"}],\"packageUris\":[\"http://schema.mathworks.com/mf0/Connector/R2020b\"],\"version\":\"1.0\"}"
      mask TypeOptions popup_driveJointF: CV Joint | U Joint
      mask TypeOptions popup_driveJointR: CV Joint | U Joint
  Ground Contact FL : wheel_loader_contact_lib/Ground Contact Tire  VariantControl=Choice  LabelModeActiveChoice=Sphere  popup_contact=Sphere  ptcld_xyz=HMPST.Tire.ptcld.FL
  Ground Contact FR : wheel_loader_contact_lib/Ground Contact Tire  VariantControl=Choice  LabelModeActiveChoice=Sphere  popup_contact=Sphere  ptcld_xyz=HMPST.Tire.ptcld.FR
  Ground Contact RL : wheel_loader_contact_lib/Ground Contact Tire  VariantControl=Choice  LabelModeActiveChoice=Sphere  popup_contact=Sphere  ptcld_xyz=HMPST.Tire.ptcld.RL
  Ground Contact RR : wheel_loader_contact_lib/Ground Contact Tire  VariantControl=Choice  LabelModeActiveChoice=Sphere  popup_contact=Sphere  ptcld_xyz=HMPST.Tire.ptcld.RR
  Wheel FL : Subsystem
      mask Display: image('sm_wheel_loader_vehicle_Wheel_IMAGE.png');
  Wheel FR : Subsystem
      mask Display: image('sm_wheel_loader_vehicle_Wheel_IMAGE.png')
  Wheel RL : Subsystem
      mask Display: image('sm_wheel_loader_vehicle_Wheel_IMAGE.png')
  Wheel RR : Subsystem
      mask Display: image('sm_wheel_loader_vehicle_Wheel_IMAGE.png')
  Tr : PMIOPort  Side=Right
  R : PMIOPort  Port=2  Side=Right
  F : PMIOPort  Port=3  Side=Right
  G : PMIOPort  Port=4  Side=Right
  Out Bus Element : Outport  PortName=m  Element=Wheel
  wires:
  Bus Creator/1 -> Out Bus Element/1
  [RR] -> Bus Creator/4  "RR"
  [RL] -> Bus Creator/3  "RL"
  [FR] -> Bus Creator/2  "FR"
  [FL] -> Bus Creator/1  "FL"
  Ground Contact RR/1 -> [RR]
  Ground Contact FR/1 -> [FR]
  Ground Contact FL/1 -> [FL]
  Ground Contact RL/1 -> [RL]
  connections:
  Tr/RConn1 -- Driveline/RConn2
  Ground Contact RL/RConn1 -- Connection Label4/LConn1
  Ground Contact RL/LConn1 -- Wheel RL/LConn1
  Ground Contact RR/RConn1 -- Connection Label3/LConn1
  Ground Contact FL/RConn1 -- Connection Label2/LConn1
  Ground Contact FR/RConn1 -- Connection Label1/LConn1
  G/RConn1 -- Connection Label/LConn1
  Ground Contact FR/LConn1 -- Wheel FR/RConn1
  Driveline/RConn3 -- Wheel FR/LConn1
  Driveline/LConn3 -- Wheel FL/RConn1
  Ground Contact FL/LConn1 -- Wheel FL/LConn1
  Driveline/LConn1 -- Wheel RL/RConn1
  Ground Contact RR/LConn1 -- Wheel RR/RConn1
  Driveline/RConn1 -- Wheel RR/LConn1
  Driveline/RConn6 -- Axle Housing Front/LConn3
  Driveline/RConn5 -- Axle Housing Front/LConn2
  Driveline/RConn4 -- Axle Housing Front/LConn1
  Driveline/LConn6 -- Axle Housing Rear/RConn3
  Driveline/LConn5 -- Axle Housing Rear/RConn2
  Driveline/LConn4 -- Axle Housing Rear/RConn1
  F/RConn1 -- Axle Housing Front/RConn1
  Axle Housing Rear/LConn1 -- R/RConn1

== system sm_wheel_loader_lib/Wheel Loader Vehicle/Frame Front ==
  Camera Frames : Subsystem
  Fender FL : Subsystem  Tag=23FC4218-D579-E34B-A76B-8575254F2127
  Fender FR : Subsystem  Tag=09759EF1-6615-2140-AB69-C7D1A2E7CB45
  FrontFrame : Subsystem  Tag=8DD4DE4B-D0E2-8341-9F65-F61D78DC0BCD
  Lights : Subsystem
  SteeringActRodBearing : Subsystem  Tag=03D27E01-1F06-D945-BD84-AA4BCEEC5D59
  Transform Lights : sm_lib/Frames and Transforms/Rigid Transform  RotationMethod=None  FollAlignAxisA=+X  BaseAlignAxisA=+Y  FollAlignAxisB=+Y  BaseAlignAxisB=+Z  RotationStandardAxis=+Z  RotationAngle=0.0  RotationAngleUnits=deg  RotationArbitraryAxis=[0 0 1]  RotationSequenceAxes=FollowerAxes  RotationSequence=XYX  RotationSequenceAngles=[0 0 0]  RotationSequenceAnglesUnits=deg  RotationMatrix=[1 0 0; 0 1 0; 0 0 1]  Quaternion=[1 0 0 0]  TranslationMethod=Cartesian  TranslationCartesianOffset=[0 0 -0.1895]  TranslationCartesianOffsetUnits=m  TranslationStandardAxis=+Z  TranslationStandardOffset=0  TranslationStandardOffsetUnits=m  TranslationROffset=0  TranslationROffsetUnits=m  TranslationThetaOffset=0  TranslationThetaOffsetUnits=deg  TranslationZOffset=0  TranslationZOffsetUnits=m
  Transform Ref : sm_lib/Frames and Transforms/Rigid Transform  RotationMethod=StandardAxis  FollAlignAxisA=+X  BaseAlignAxisA=+Y  FollAlignAxisB=+Y  BaseAlignAxisB=+Z  RotationStandardAxis=+Z  RotationAngle=90  RotationAngleUnits=deg  RotationArbitraryAxis=[0 0 1]  RotationSequenceAxes=FollowerAxes  RotationSequence=XYX  RotationSequenceAngles=[0 0 0]  RotationSequenceAnglesUnits=deg  RotationMatrix=[1 0 0; 0 1 0; 0 0 1]  Quaternion=[1 0 0 0]  TranslationMethod=Cartesian  TranslationCartesianOffset=[0 0.8705 -0.69773+0.1143]  TranslationCartesianOffsetUnits=m  TranslationStandardAxis=+Z  TranslationStandardOffset=0  TranslationStandardOffsetUnits=m  TranslationROffset=0  TranslationROffsetUnits=m  TranslationThetaOffset=0  TranslationThetaOffsetUnits=deg  TranslationZOffset=0  TranslationZOffsetUnits=m
  Steer : PMIOPort  Side=Left
  Hinge : PMIOPort  Port=2  Side=Left
  LiftL : PMIOPort  Port=3  Side=Right
  LiftR : PMIOPort  Port=4  Side=Right
  Tilt : PMIOPort  Port=5  Side=Right
  Arm : PMIOPort  Port=6  Side=Right
  Drive : PMIOPort  Port=7  Side=Left
  Ref : PMIOPort  Port=8  Side=Right
  connections:
  Lights/LConn1 -- Transform Lights/RConn1
  FrontFrame/RConn3 -- LiftR/RConn1
  Steer/RConn1 -- FrontFrame/LConn1
  Fender FL/LConn1 -- FrontFrame/RConn7
  FrontFrame/RConn2 -- LiftL/RConn1
  Fender FR/LConn1 -- FrontFrame/RConn8
  SteeringActRodBearing/LConn1 -- FrontFrame/RConn1
  FrontFrame/RConn6 -- Drive/RConn1
  FrontFrame/RConn5 -- Arm/RConn1
  FrontFrame/RConn4 -- Tilt/RConn1
  Hinge/RConn1 -- Transform Ref/LConn1 -- Camera Frames/LConn1 -- Transform Lights/LConn1 -- FrontFrame/LConn2
  Ref/RConn1 -- Transform Ref/RConn1

== system sm_wheel_loader_lib/Wheel Loader Vehicle/Frame Rear ==
  BusElementIn : Inport  PortName=Cmd
  Bus Selector : BusSelector  OutputSignals=Operator.SteerCmd
  Cab : Subsystem  Tag=8AB14510-8440-2D42-A5EA-732CCF7C6FFF
  Camera Frames : Subsystem
  Chassis : Subsystem  Tag=0034DD1C-3F78-EA48-8EB0-FD1E79A95281
  Counterweight : Subsystem  Tag=99BCECF5-04B2-334D-A294-C62C2B495A17
  Damper Steering : fl_lib/Mechanical/Rotational Elements/Rotational Damper  D=0.001 N*m*s/rad  w_specify=off  w_priority=None  w=0 rad/s  w_nominal_specify=off  w_nominal_value=1  w_nominal_unit=rad/s  t_specify=off  t_priority=None  t=0 N*m  t_nominal_specify=off  t_nominal_value=1  t_nominal_unit=N*m
  Fender RL : Subsystem  Tag=D7356064-A80E-C343-BF50-4E22E2FDD7AB
  Fender RR : Subsystem  Tag=9CFF811C-0389-C14E-A239-3CC5CD817F6B
  Handles Panels : Subsystem
  Hood : Subsystem  Tag=528F8BEE-8CB9-ED45-8BD2-87AC8441592E
  Mechanical Rotational Reference : fl_lib/Mechanical/Rotational Elements/Mechanical Rotational Reference
  Reference Frame : sm_lib/Frames and Transforms/Reference Frame
  Revolute Steer : sm_lib/Joints/Revolute Joint  JointMode=Normal  CompositeWrenchDir=FollowerOnBase  CompositeWrenchFrame=BaseFrame  SenseConstraintForce=off  SenseConstraintTorque=off  SenseTotalForce=off  SenseTotalTorque=off  PositionTargetSpecify=off  PositionTargetPriority=High  PositionTargetValue=0  PositionTargetValueUnits=deg  VelocityTargetSpecify=off  VelocityTargetPriority=High  VelocityTargetValue=0  VelocityTargetValueUnits=deg/s  EquilibriumPosition=0  EquilibriumPositionUnits=deg  SpringStiffness=0  SpringStiffnessUnits=N*m/deg  DampingCoefficient=0  DampingCoefficientUnits=N*m/(deg/s)  LowerLimitSpecify=off  LowerLimitBound=-90  LowerLimitBoundUnits=deg  LowerLimitStiffness=1e4  LowerLimitStiffnessUnits=N*m/deg  LowerLimitDamping=10  LowerLimitDampingUnits=N*m/(deg/s)  LowerLimitTransitionRegionWidth=0.1  LowerLimitTransitionRegionWidthUnits=deg  UpperLimitSpecify=off  UpperLimitBound=90  UpperLimitBoundUnits=deg  UpperLimitStiffness=1e4  UpperLimitStiffnessUnits=N*m/deg  UpperLimitDamping=10  UpperLimitDampingUnits=N*m/(deg/s)  UpperLimitTransitionRegionWidth=0.1  UpperLimitTransitionRegionWidthUnits=deg  TorqueActuationMode=ComputedTorque  MotionActuationMode=InputMotion  SensePosition=off  SenseVelocity=on  SenseAcceleration=off  SenseTorqueForce=off  SenseLowerLimitTorqueForce=off  SenseUpperLimitTorqueForce=off
  Rigid Transform : sm_lib/Frames and Transforms/Rigid Transform  RotationMethod=StandardAxis  FollAlignAxisA=+X  BaseAlignAxisA=+Y  FollAlignAxisB=+Y  BaseAlignAxisB=+Z  RotationStandardAxis=+X  RotationAngle=-25  RotationAngleUnits=deg  RotationArbitraryAxis=[0 0 1]  RotationSequenceAxes=FollowerAxes  RotationSequence=XYX  RotationSequenceAngles=[0 0 0]  RotationSequenceAnglesUnits=deg  RotationMatrix=[1 0 0;0 1 0;0 0 1]  Quaternion=[1 0 0 0]  TranslationMethod=Cartesian  TranslationCartesianOffset=[0 0.25 0.45]  TranslationCartesianOffsetUnits=m  TranslationStandardAxis=+Z  TranslationStandardOffset=0  TranslationStandardOffsetUnits=m  TranslationROffset=0  TranslationROffsetUnits=m  TranslationThetaOffset=0  TranslationThetaOffsetUnits=deg  TranslationZOffset=0  TranslationZOffsetUnits=m
  Simulink-PS Converter : nesl_utility/Simulink-PS Converter  PhysicalDomain=network_engine_domain  SubClassName=ps_input  LeftPortType=input  RightPortType=output  PseudoPeriodic=off  Frequencies=[]  NoiseDistribution=none  NoiseParameters=[]  Unit=rad  AffineConversion=off  FilteringAndDerivatives=filter  SimscapeFilterOrder=2  InputFilterTimeConstant=0.01  UdotUserProvided=0
  Steering Wheel : Subsystem
  SteeringActCylBearing : Subsystem  Tag=3B841C06-DAE6-6448-91C4-4496AD0D8B5F
  SteeringCoupler : Subsystem  Tag=2E9E311A-265F-DD4B-8FE4-6B9B9F7FC7AE
  Transform Handles : sm_lib/Frames and Transforms/Rigid Transform  RotationMethod=None  FollAlignAxisA=+X  BaseAlignAxisA=+Y  FollAlignAxisB=+Y  BaseAlignAxisB=+Z  RotationStandardAxis=+Z  RotationAngle=0.0  RotationAngleUnits=deg  RotationArbitraryAxis=[0 0 1]  RotationSequenceAxes=FollowerAxes  RotationSequence=XYX  RotationSequenceAngles=[0 0 0]  RotationSequenceAnglesUnits=deg  RotationMatrix=[1 0 0; 0 1 0; 0 0 1]  Quaternion=[1 0 0 0]  TranslationMethod=Cartesian  TranslationCartesianOffset=[0 0 -0.1895]  TranslationCartesianOffsetUnits=m  TranslationStandardAxis=+Z  TranslationStandardOffset=0  TranslationStandardOffsetUnits=m  TranslationROffset=0  TranslationROffsetUnits=m  TranslationThetaOffset=0  TranslationThetaOffsetUnits=deg  TranslationZOffset=0  TranslationZOffsetUnits=m
  Velocity Source Steering Wheel : fl_lib/Mechanical/Mechanical Sources/Ideal Angular Velocity Source
  Steer : PMIOPort  Side=Right
  Hinge : PMIOPort  Port=2  Side=Right
  Drive : PMIOPort  Port=3  Side=Right
  S : PMIOPort  Port=4  Side=Left
  wires:
  BusElementIn/1 -> Bus Selector/1
  Bus Selector/1 -> Simulink-PS Converter/1  "<SteerCmd>"
  connections:
  Handles Panels/LConn1 -- Transform Handles/RConn1
  Hinge/RConn1 -- Transform Handles/LConn1 -- Camera Frames/LConn1 -- Chassis/RConn4
  Chassis/RConn2 -- SteeringActCylBearing/LConn1
  Cab/RConn1 -- Hood/LConn1
  SteeringCoupler/LConn1 -- Chassis/RConn3
  Cab/LConn1 -- Chassis/RConn5
  Reference Frame/RConn1 -- Chassis/LConn1
  Chassis/RConn8 -- Fender RR/LConn1
  Chassis/RConn9 -- Fender RL/LConn1
  Counterweight/LConn1 -- Chassis/RConn6
  Chassis/RConn7 -- Drive/RConn1
  Chassis/RConn1 -- Steer/RConn1
  Rigid Transform/LConn1 -- Cab/RConn2
  Revolute Steer/LConn1 -- Rigid Transform/RConn1
  Revolute Steer/RConn1 -- Steering Wheel/LConn1
  Simulink-PS Converter/RConn1 -- Revolute Steer/LConn2
  Revolute Steer/RConn2 -- Velocity Source Steering Wheel/RConn1
  Damper Steering/RConn1 -- Velocity Source Steering Wheel/RConn2 -- Mechanical Rotational Reference/LConn1
  Velocity Source Steering Wheel/LConn1 -- S/RConn1 -- Damper Steering/LConn1
